simulink model "MultiRotorLowFidelity"  (R2024a)
settings: Solver=VariableStepAuto  StartTime=0.0  StopTime=10.0  RelTol=1e-3
undefined symbols (not defined in the file): Pitch, Roll, Thrust, YawRate
libraries: robotcorelib x1, uavalgslib x1, uavutilslib x1
settings Model: Creator=hrish  LastModifiedBy=hrish
settings RTWCC: GPUComputeCapability=3.5

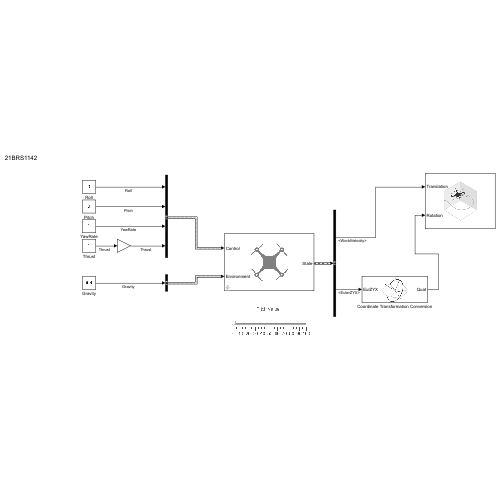
[thumbnail: Simulink's stored preview of the top-level diagram]
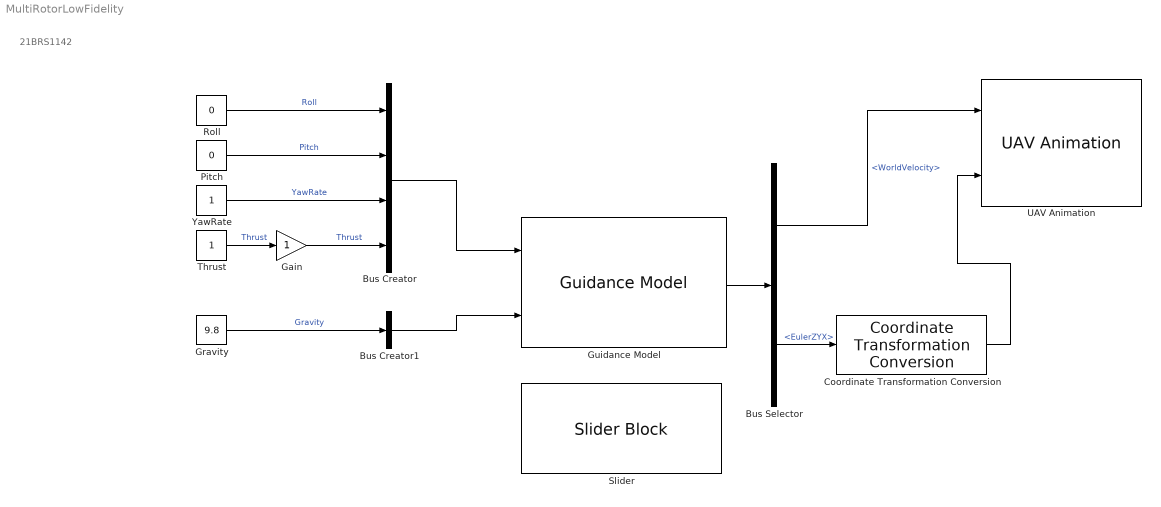
== system MultiRotorLowFidelity ==
  note: 21BRS1142
  Bus Creator : BusCreator  Inputs=Roll,Pitch,YawRate,Thrust  OutDataTypeStr=Bus: MultirotorGuidanceControlBus  NonVirtualBus=on
  Bus Creator1 : BusCreator  Inputs=Gravity  OutDataTypeStr=Bus: MultirotorGuidanceEnvironmentBus  NonVirtualBus=on
  Bus Selector : BusSelector  OutputSignals=WorldVelocity,EulerZYX
  Coordinate Transformation Conversion : robotcorelib/Coordinate Transformation Conversion  InputRepresentation=Euler Angles  InputEulerSequence=ZYX  ShowTrVecInputPort=on  OutputRepresentation=Quaternion  OutputEulerSequence=ZYX  ShowTrVecOutputPort=on  SimulateUsing=Interpreted execution
      settings: LibrarySourceBlock=uavutilslib/Coordinate Transformation Conversion
  Gain : Gain
  Gravity : Constant  Value=9.8
  Guidance Model : uavalgslib/Guidance Model  ModelType=MultirotorGuidance  SpecifiedDataType=double  SimulateUsing=Interpreted execution  InitialWorldPositionMultirotor=[0; 0; 0]  InitialWorldVelocityMultirotor=[0; 0; 0]  InitialEulerZYXMultirotor=[0; 0; 0]  InitialBodyAngularRateRPYMultirotor=[0; 0; 0]  InitialThrustMultirotor=0  InitialNorthFixedWing=0  InitialEastFixedWing=0  InitialHeightFixedWing=0  InitialAirSpeedFixedWing=0  InitialHeadingAngleFixedWing=0  InitialFlightPathAngleFixedWing=0  InitialRollAngleFixedWing=0  InitialRollAngleRateFixedWing=0  PDRollMultirotor=[3402.97,116.67]  PDPitchMultirotor=[3402.97, 116.67]  PYawRateMultirotor=1950  PThrustMultirotor=3900  MassMultirotor=0.1  PHeightFixedWing=3.9  PHeadingAngleFixedWing=3.9  PFlightPathAngleFixedWing=39  PDRollFixedWing=[3402.97, 116.67]  PAirSpeedFixedWing=1  FlightPathAngleLimitsFixedWing=[-pi/2, pi/2]  StateBusName='MultirotorGuidanceStateBus'  ControlBusName='MultirotorGuidanceControlBus'  EnvironmentBusName='MultirotorGuidanceEnvironmentBus'  DataType=double
  Pitch : Constant  Value=0
  Roll : Constant  Value=0
  Slider : SliderBlock
  Thrust : Constant
  UAV Animation : uavutilslib/UAV Animation  UAVType=Multirotor  UAVSize=1  InertialZDirection=Down  SampleTime=-1
  YawRate : Constant
  wires:
  Roll/1 -> Bus Creator/1  "Roll"
  Pitch/1 -> Bus Creator/2  "Pitch"
  YawRate/1 -> Bus Creator/3  "YawRate"
  Thrust/1 -> Gain/1  "Thrust"
  Gain/1 -> Bus Creator/4  "Thrust"
  Bus Creator/1 -> Guidance Model/1
  Gravity/1 -> Bus Creator1/1  "Gravity"
  Bus Creator1/1 -> Guidance Model/2
  Guidance Model/1 -> Bus Selector/1
  Bus Selector/2 -> Coordinate Transformation Conversion/1  "<EulerZYX>"
  Coordinate Transformation Conversion/1 -> UAV Animation/2
  Bus Selector/1 -> UAV Animation/1  "<WorldVelocity>"
